simulink model "alg_loop_after_compiling"  (R2015a)
settings: Solver=ode45  StartTime=0.0  StopTime=10.0  RelTol=1e-3
libraries: simulink x3
settings Model: Creator=shafiul  LastModifiedBy=shafiul

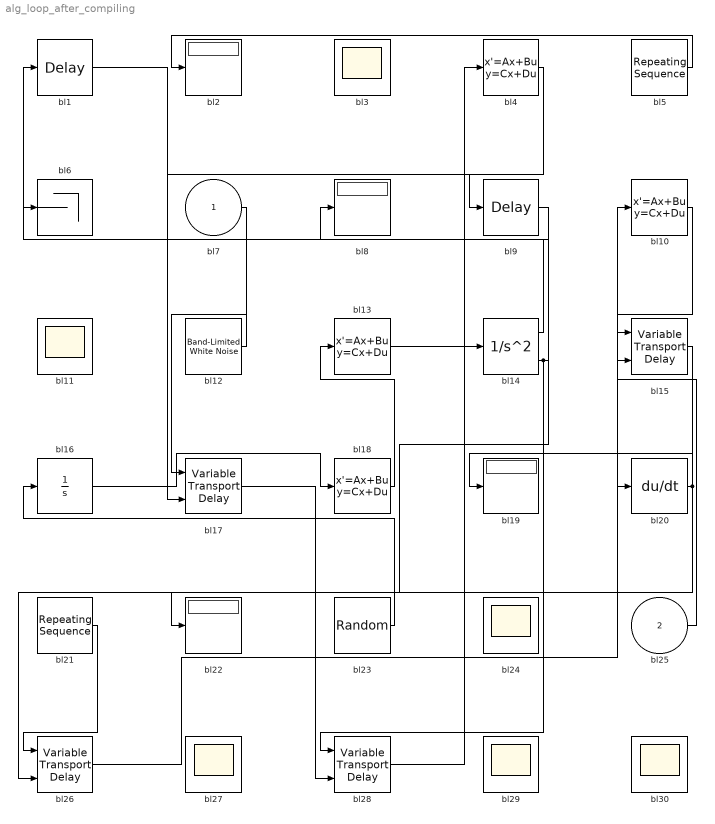
== system alg_loop_after_compiling ==
  bl7 : Inport
  bl25 : Inport  Port=2
  bl1 : TransportDelay  InitialOutput=1
  bl{4,10,13,18} (4 alike) : StateSpace  X0=0
  bl{3,11,24,27,29..30} (6 alike) : Scope
      settings: Floating=on
  bl12 : simulink/Sources/Band-Limited White Noise  Cov=[0.1]  Ts=0.1  seed=[23341]
  bl14 : SecondOrderIntegrator  LimitX=on  UpperLimitX=1  LowerLimitX=0  LimitDXDT=on
  bl15 : VariableTransportDelay  MaximumDelay=10  InitialOutput=1  ZeroDelay=on
  bl16 : Integrator
  bl17 : VariableTransportDelay  MaximumDelay=10  InitialOutput=3  ZeroDelay=on
  bl{2,8,19,22} (4 alike) : Display
  bl20 : Derivative
  bl21 : simulink/Sources/Repeating Sequence  rep_seq_t=[0 2]  rep_seq_y=[0 2]
  bl23 : RandomNumber  SampleTime=0.1
  bl26 : VariableTransportDelay  MaximumDelay=10  InitialOutput=3  ZeroDelay=on
  bl28 : VariableTransportDelay  MaximumDelay=10  InitialOutput=1  ZeroDelay=on
  bl5 : simulink/Sources/Repeating Sequence  rep_seq_t=[0 2]  rep_seq_y=[0 2]
  bl6 : Terminator
  bl9 : TransportDelay  InitialOutput=1
  wires:
  bl26/1 -> bl10/1
  bl14/1 -> bl1/1
  bl13/1 -> bl14/1
  bl10/1 -> bl20/1
  bl15/1 -> bl19/1
  bl5/1 -> bl2/1
  bl16/1 -> bl18/1
  bl12/1 -> bl6/1
  bl7/1 -> bl17/1
  bl9/1 -> bl22/1
  bl14/2 -> bl28/1, bl8/1
  bl4/1 -> bl17/2
  bl1/1 -> bl9/1
  bl23/1 -> bl16/1
  bl20/1 -> bl15/1, bl26/2
  bl25/1 -> bl15/2
  bl21/1 -> bl26/1
  bl17/1 -> bl28/2
  bl18/1 -> bl13/1
  bl28/1 -> bl4/1
